simulink model "LMS_cs_old"  (R2023a)
settings: Solver=ode5  StartTime=0.0  StopTime=inf  FixedStep=1/200  RelTol=1e-3
PreLoadFcn:
  | mbxruntime.callbacks.PreLoadFcn(bdroot);
PostLoadFcn:
  | mbxruntime.callbacks.PostLoadFcn(bdroot);
InitFcn:
  | mbxruntime.callbacks.InitFcn(bdroot);
StartFcn:
  | mbxruntime.callbacks.StartFcn(bdroot);
StopFcn:
  | mbxruntime.callbacks.StopFcn(bdroot);
model workspace (MAT data in the model file):
  mbox_table : object (value not decoded)
  model_closed = 0
  sim_status = 0
undefined symbols (not defined in the file or in its folder): DiscIntNeverNeededParam, WheelL0, WheelL1, WheelR0, WheelR1
libraries: simulink x462, simulink_extras x117, PreScanSimulinkLibrary x33, PreScanUsefulBlocks x6, instrumentseriallib x5, simulink_need_slupdate x1
(part 10 of 68)

== system LMS_cs_old/BMW_X5_SUV_4/Dynamics_Simple_3D ==
  DeltaSteer_[deg] : Inport
  Throttle : Inport  Port=2
  Brake : Inport  Port=3
  Initial_Vx_[ms-1] : Inport  Port=4
  AutoManual_OnOff : Inport  Port=5
  Auto_GearShift : Inport  Port=6
  Manual_GearShift : Inport  Port=7
  TyreInfo_in : Inport  Port=8
  Bus Creator : BusCreator  Inputs=14
  Bus Selector : BusSelector  OutputSignals=z_wheelFL_[m],z_wheelFR_[m],z_wheelRL_[m],z_wheelRR_[m]
  Chassis : Subsystem
      mask Display: image(imread('Chassis.png'));
  Engine : Subsystem
      mask Display: image(imread('Engine.png'));
  Gain : Gain  Gain=3.6
  Gear: Auto Manual : Subsystem
  Mux : Mux  Inputs=3
  Radians to Degrees : simulink_extras/Transformations/Radians to Degrees
  Radians to Degrees1 : simulink_extras/Transformations/Radians to Degrees
  Selector : Selector  InputPortWidth=9  IndexOptions=Index vector (dialog)  Indices=7  OutputSizes=1
  Selector1 : Selector  InputPortWidth=9  IndexOptions=Index vector (dialog)  Indices=8  OutputSizes=1
  ShiftLogic : Subsystem
      mask Display: image(imread('Gearshift.png'));
  Transmission : Subsystem
      mask Display: image(imread('Transmission.png'));
  State : Outport
  Vx [m s-1] : Outport  Port=2
  Perf_Params : Outport  Port=3
  z_wheelFL_[m] : Outport  Port=4
  z_wheelFR_[m] : Outport  Port=5
  z_wheelRL_[m] : Outport  Port=6
  z_wheelRR_[m] : Outport  Port=7
  ContactParams : Outport  Port=8
  wires:
  [ax] -> Bus Creator/4  "Ax_[ms-2]"
  [vx] -> Gain/1
  Selector1/1 -> Radians to Degrees1/1
  Selector/1 -> Radians to Degrees/1
  [PD] -> Bus Creator/10  "PDrive_[kW]"
  Radians to Degrees1/1 -> Bus Creator/12  "Pitch_[deg]"
  Radians to Degrees/1 -> Bus Creator/11  "Roll_[deg]"
  [PE] -> Bus Creator/9  "PEngine_[kW]"
  Bus Creator/1 -> Perf_Params/1
  Engine/2(PEngine_[kW]) -> [PE]
  [brake] -> Bus Creator/8  "Brake_[bar]"
  [throttle] -> Bus Creator/7  "Throttle_[perc]"
  [auto_manual] -> Bus Creator/6  "Auto_Manual_[-]"
  [ay] -> Bus Creator/5  "Ay_[ms-2]"
  [gear] -> Bus Creator/3  "Gear_[-]"
  [RPM] -> Bus Creator/2  "NEngine_[rpm]"
  Gain/1 -> Bus Creator/1  "Vx_[kmh-1]"
  Transmission/1(ImpellerTorque_[Nm]) -> Engine/1(ImpellerTorque_[Nm])  "ImpellerTorque_[Nm]"
  Transmission/2(TransmissionTorque_[Nm]) -> Chassis/1(TransmissionTorque_[Nm])  "TransmissionTorque_[Nm]"
  ShiftLogic/1(GearNr) -> ShiftLogic/2(GearNr_[-]), Gear: Auto Manual/3(Auto_Gear)  "GearNr_[-]"
  Engine/1(nEngine_[rpm]) -> Transmission/1(nEngine_[rpm]), [RPM]  "nEngine_[rpm]"
  Chassis/1(State) -> Selector1/1, Selector/1, State/1, Mux/1
  DeltaSteer_[deg]/1 -> Chassis/3(DeltaSteer_[deg])
  Initial_Vx_[ms-1]/1 -> Chassis/4(Initial_Vx_[ms-1])
  Throttle/1 -> [throttle], ShiftLogic/1(Throttle_[%]), Engine/2(Throttle_[%])
  Auto_GearShift/1 -> ShiftLogic/3(Auto_GearShift)
  Chassis/7(TransmissionOut_[rpm]) -> Transmission/3(n_TransmissionOut_[rpm])  "n_driveline_[rpm]"
  Chassis/2(VehicleSpeed_[ms-1]) -> [vx], Vx [m s-1]/1, Mux/2  "vx_[ms-1]"
  AutoManual_OnOff/1 -> [auto_manual], Gear: Auto Manual/1(Auto_Manual)
  Manual_GearShift/1 -> Gear: Auto Manual/2(Manual_Gear)
  Gear: Auto Manual/1(Gear) -> [gear], Transmission/2(GearNr_[-])  "gear"
  [vx] -> ShiftLogic/4(VehSpeed_[ms-1])
  TyreInfo_in/1 -> Chassis/5(TyreInfo_in)
  Brake/1 -> Chassis/2(BrakePressure_[bar]), [brake]
  Chassis/6(PDrive_[kW]) -> [PD]
  Chassis/5(ay_[ms-2]) -> [ay]
  Chassis/4(ax_[ms-2]) -> [ax]
  Chassis/3(Vy_[ms-1]) -> [vy]
  [vx] -> Bus Creator/13  "vx_[ms-1]"
  [vy] -> Bus Creator/14  "vy_[ms-1]"
  Chassis/8(z_wheel_[m]) -> Bus Selector/1, Mux/3  "z_wheel_[m]"
  Bus Selector/1 -> z_wheelFL_[m]/1  "<z_wheelFL_[m]>"
  Bus Selector/2 -> z_wheelFR_[m]/1  "<z_wheelFR_[m]>"
  Bus Selector/3 -> z_wheelRL_[m]/1  "<z_wheelRL_[m]>"
  Bus Selector/4 -> z_wheelRR_[m]/1  "<z_wheelRR_[m]>"
  Mux/1 -> ContactParams/1

== system LMS_cs_old/BMW_X5_SUV_4/JointGroup_WheelDisplacement_V2R ==
  Velocity [m/s] : Inport  SampleTime=TimeStep
  Discrete-Time Integrator : DiscreteIntegrator  SampleTime=TimeStep  ICPrevOutput=DiscIntNeverNeededParam  ICPrevScaledInput=DiscIntNeverNeededParam
  omega=V/Rwheel : Gain  Gain=1/TireRadius
  Rotation [rad] : Outport
  wires:
  Discrete-Time Integrator/1 -> Rotation [rad]/1  "roty"
  omega=V/Rwheel/1 -> Discrete-Time Integrator/1  "rotational speed [rad/s]"
  Velocity [m/s]/1 -> omega=V/Rwheel/1

== system LMS_cs_old/BMW_X5_SUV_4/PreScan_Contact_Sensor ==
  ContactParams : Inport  SampleTime=TimeStep
  Steer Angle Front [deg] : Inport  Port=2
  Steer Angle Rear [deg] : Inport  Port=3
  Bus Creator2 : BusCreator  Inputs=4
  Demux : Demux
  Demux1 : Demux  Outputs=[9 1 4]
  Demux2 : Demux
  For All Wheel Contacts : Subsystem  TreatAsAtomicUnit=on
  Mux6 : Mux  Inputs=2
  Subsystem : Subsystem  mask{NumberOfWheels=4, MaxContactPoints=4, WheelRadius=wheelRadius, WheelWidth=0.2}
      mask prompts: NumberOfWheels "Number of Wheels"; MaxContactPoints "Maximum number of Contact Points"; WheelRadius "Wheel Radius"; WheelWidth "Wheel Width"
      mask Display: disp('Contact Sensor')
  Tire Collision Demux : Subsystem
  Tire Collision Demux1 : Subsystem
  Tire Collision Demux2 : Subsystem
  Tire Collision Demux3 : Subsystem
  Vehicle Local to World : Subsystem
  Wheels = 4 : Subsystem  mask{NumberOfWheels=4}
      mask prompts: NumberOfWheels "Number of Wheels"
      mask Display:
      | port_label('input', 1,'Vehicle wrt World')
      | port_label('input', 2,'Wheels wrt World')
  Wheels Local to World : Subsystem  Tag=MuxWheels  mask(PreScan Mux Block:){}
      settings: DeleteFcn=PreScanBlockDeleteFcn;
  Results : Outport
  wires:
  Mux6/1 -> Wheels = 4/1(Vehicle wrt World)
  Wheels = 4/1(WheelPoses) -> Subsystem/1(In1)
  Demux/1 -> Tire Collision Demux/1(demux in)
  Demux/2 -> Tire Collision Demux1/1(demux in)
  Demux/3 -> Tire Collision Demux2/1(demux in)
  Demux/4 -> Tire Collision Demux3/1(demux in)
  Tire Collision Demux/1(bus out) -> Bus Creator2/1  "TireFL"
  Tire Collision Demux1/1(bus out) -> Bus Creator2/2  "TireFR"
  Tire Collision Demux2/1(bus out) -> Bus Creator2/3  "TireRL"
  Tire Collision Demux3/1(bus out) -> Bus Creator2/4  "TireRR"
  Vehicle Local to World/1(Position) -> Mux6/1
  Vehicle Local to World/2(Orientation) -> Mux6/2
  Wheels Local to World/1(Wheel Poses) -> Wheels = 4/2(Wheels wrt World)
  Demux1/2 -> Wheels Local to World/3(Velocity [m/s])
  Demux2/1 -> Wheels Local to World/4(zDisp FL [m])
  Demux2/2 -> Wheels Local to World/5(zDisp FR [m])
  Demux2/3 -> Wheels Local to World/6(zDisp RL [m])
  Demux2/4 -> Wheels Local to World/7(zDisp RR [m])
  Steer Angle Front [deg]/1 -> Wheels Local to World/1(Steer Angle Front [deg])
  Steer Angle Rear [deg]/1 -> Wheels Local to World/2(Steer Angle Rear [deg])
  Bus Creator2/1 -> Results/1
  ContactParams/1 -> Demux1/1
  Demux1/1 -> Vehicle Local to World/1(State)
  Demux1/3 -> Demux2/1
  Subsystem/1(Out1) -> For All Wheel Contacts/1(In1)
  For All Wheel Contacts/1(Out1) -> Demux/1

== system LMS_cs_old/BMW_X5_SUV_4/SELF_Demux ==
  SELF : Inport  OutDataTypeStr=Bus: PRESCAN_SELFSENSORDATA
  Bus Selector : BusSelector  OutputSignals=PositionX,PositionY,PositionZ,OrientationRoll,OrientationPitch,OrientationYaw,Velocity,Yaw_rate,Lat,Long,Alt
  Demux2 : Demux  Outputs=3
  Gain : Gain  Gain=180/pi
  Gain1 : Gain  Gain=180/pi
  Vector Concatenate1 : Concatenate  NumInputs=3
  compas converter : Subsystem
  x [m] : Outport
  y [m] : Outport  Port=2
  z [m] : Outport  Port=3
  rotx [deg] : Outport  Port=4
  roty [deg] : Outport  Port=5
  rotz [deg] : Outport  Port=6
  GPS lat [deg] : Outport  Port=7
  GPS long [deg] : Outport  Port=8
  GPS alt [m] : Outport  Port=9
  velocity [m/s] : Outport  Port=10
  heading [deg] : Outport  Port=11
  yaw rate [deg/s] : Outport  Port=12
  wires:
  Bus Selector/11 -> GPS alt [m]/1  "<Alt>"
  Bus Selector/10 -> GPS long [deg]/1  "<Long>"
  Bus Selector/9 -> GPS lat [deg]/1  "<Lat>"
  Bus Selector/8 -> Gain1/1  "<Yaw_rate>"
  Bus Selector/7 -> velocity [m/s]/1  "<Velocity>"
  Bus Selector/6 -> compas converter/1(rotz [rad]), Vector Concatenate1/3  "<OrientationYaw>"
  Bus Selector/5 -> Vector Concatenate1/2  "<OrientationPitch>"
  Bus Selector/4 -> Vector Concatenate1/1  "<OrientationRoll>"
  Vector Concatenate1/1 -> Gain/1
  Bus Selector/3 -> z [m]/1  "<PositionZ>"
  Bus Selector/2 -> y [m]/1  "<PositionY>"
  Bus Selector/1 -> x [m]/1  "<PositionX>"
  SELF/1 -> Bus Selector/1
  Gain/1 -> Demux2/1
  Demux2/1 -> rotx [deg]/1
  Demux2/2 -> roty [deg]/1
  Demux2/3 -> rotz [deg]/1
  compas converter/1(heading [deg]) -> heading [deg]/1
  Gain1/1 -> yaw rate [deg/s]/1

== system LMS_cs_old/BMW_X5_SUV_4/STATE_BMW_X5_SUV_4 ==
  State : Inport  SampleTime=TimeStep
  Bus Creator : BusCreator  Inputs=15  OutDataTypeStr=Bus: PRESCAN_STATEACTUATORDATA  NonVirtualBus=on
  Demux : Demux  Outputs=15
  iniBODYAngles wrtVEH [rad] : Constant  Value=[Roll0 Pitch0 0]  SampleTime=TimeStep
  iniVEHAngles wrtGLOB [rad] : Constant  Value=[0 0 Yaw0]  SampleTime=TimeStep
  iniVEHposition wrtGLOB [m] : Constant  Value=[x0 y0 z0]  SampleTime=TimeStep
  state2FullState : PreScanSimulinkLibrary/state2FullState  SystemSampleTime=-1  VariantActivationTime=update diagram  Latency=0  AutoFrameSizeCalculation=off
  StateBus : Outport  OutDataTypeStr=Bus: PRESCAN_STATEACTUATORDATA
  wires:
  Bus Creator/1 -> StateBus/1
  State/1 -> state2FullState/1
  state2FullState/1 -> Demux/1
  iniVEHposition wrtGLOB [m]/1 -> state2FullState/2
  iniBODYAngles wrtVEH [rad]/1 -> state2FullState/3
  iniVEHAngles wrtGLOB [rad]/1 -> state2FullState/4
  Demux/1 -> Bus Creator/1  "PositionX"
  Demux/2 -> Bus Creator/2  "PositionY"
  Demux/3 -> Bus Creator/3  "PositionZ"
  Demux/4 -> Bus Creator/4  "VelocityX"
  Demux/5 -> Bus Creator/5  "VelocityY"
  Demux/6 -> Bus Creator/6  "VelocityZ"
  Demux/7 -> Bus Creator/7  "AccelerationX"
  Demux/8 -> Bus Creator/8  "AccelerationY"
  Demux/9 -> Bus Creator/9  "AccelerationZ"
  Demux/10 -> Bus Creator/10  "OrientationRoll"
  Demux/11 -> Bus Creator/11  "OrientationPitch"
  Demux/12 -> Bus Creator/12  "OrientationYaw"
  Demux/13 -> Bus Creator/13  "AngularVelocityRoll"
  Demux/14 -> Bus Creator/14  "AngularVelocityPitch"
  Demux/15 -> Bus Creator/15  "AngularVelocityYaw"

== system LMS_cs_old/BMW_X5_SUV_4/WheelDisplacement_Mux ==
  Steering Angle Front [rad] : Inport  Tag=inport/JointGroup  SampleTime=2/200  BusOutputAsStruct=on
  Steering Angle Rear [rad] : Inport  Tag=inport/JointGroup  Port=2  SampleTime=2/200  BusOutputAsStruct=on
  Rotation [rad] : Inport  Tag=inport/JointGroup  Port=3  SampleTime=2/200  BusOutputAsStruct=on
  zDisp FL [m] : Inport  Tag=inport/JointGroup  Port=4  SampleTime=2/200  BusOutputAsStruct=on
  zDisp FR [m] : Inport  Tag=inport/JointGroup  Port=5  SampleTime=2/200  BusOutputAsStruct=on
  zDisp RL [m] : Inport  Tag=inport/JointGroup  Port=6  SampleTime=2/200  BusOutputAsStruct=on
  zDisp RR [m] : Inport  Tag=inport/JointGroup  Port=7  SampleTime=2/200  BusOutputAsStruct=on
  Ground_{1..12} (12 alike) : Ground
  WheelL0_Mux : Subsystem  Tag=mux/Joint  mask(PreScan Mux Block){DisplayName=WheelL0}
      mask prompts: DisplayName "Display Name"
      mask help:
      | This block simulates a generic joint used for generic models. This joint can be enabled/disabled from the GUI.
      |
      | For more information, please click Help.
      settings: DeleteFcn=PreScanBlockDeleteFcn;
      mask Help: eval('openHelp(254)')
  WheelL1_Mux : Subsystem  Tag=mux/Joint  mask(PreScan Mux Block){DisplayName=WheelL1}
      mask prompts: DisplayName "Display Name"
      mask help:
      | This block simulates a generic joint used for generic models. This joint can be enabled/disabled from the GUI.
      |
      | For more information, please click Help.
      settings: DeleteFcn=PreScanBlockDeleteFcn;
      mask Help: eval('openHelp(254)')
  WheelR0_Mux : Subsystem  Tag=mux/Joint  mask(PreScan Mux Block){DisplayName=WheelR0}
      mask prompts: DisplayName "Display Name"
      mask help:
      | This block simulates a generic joint used for generic models. This joint can be enabled/disabled from the GUI.
      |
      | For more information, please click Help.
      settings: DeleteFcn=PreScanBlockDeleteFcn;
      mask Help: eval('openHelp(254)')
  WheelR1_Mux : Subsystem  Tag=mux/Joint  mask(PreScan Mux Block){DisplayName=WheelR1}
      mask prompts: DisplayName "Display Name"
      mask help:
      | This block simulates a generic joint used for generic models. This joint can be enabled/disabled from the GUI.
      |
      | For more information, please click Help.
      settings: DeleteFcn=PreScanBlockDeleteFcn;
      mask Help: eval('openHelp(254)')
  WheelL0_BMW_X5_SUV_4 : Outport  Tag=outport/JointActuator  OutDataTypeStr=Bus: PRESCAN_POSE_DATA  SampleTime=2/200
  WheelR0_BMW_X5_SUV_4 : Outport  Tag=outport/JointActuator  Port=2  OutDataTypeStr=Bus: PRESCAN_POSE_DATA  SampleTime=2/200
  WheelR1_BMW_X5_SUV_4 : Outport  Tag=outport/JointActuator  Port=3  OutDataTypeStr=Bus: PRESCAN_POSE_DATA  SampleTime=2/200
  WheelL1_BMW_X5_SUV_4 : Outport  Tag=outport/JointActuator  Port=4  OutDataTypeStr=Bus: PRESCAN_POSE_DATA  SampleTime=2/200
  wires:
  WheelL0_Mux/1(Joint) -> WheelL0_BMW_X5_SUV_4/1
  WheelR0_Mux/1(Joint) -> WheelR0_BMW_X5_SUV_4/1
  WheelR1_Mux/1(Joint) -> WheelR1_BMW_X5_SUV_4/1
  WheelL1_Mux/1(Joint) -> WheelL1_BMW_X5_SUV_4/1
  Steering Angle Front [rad]/1 -> WheelR0_Mux/6(Yaw [rad]), WheelL0_Mux/6(Yaw [rad])
  Steering Angle Rear [rad]/1 -> WheelR1_Mux/6(Yaw [rad]), WheelL1_Mux/6(Yaw [rad])
  Rotation [rad]/1 -> WheelR0_Mux/5(Pitch [rad]), WheelL0_Mux/5(Pitch [rad]), WheelR1_Mux/5(Pitch [rad]), WheelL1_Mux/5(Pitch [rad])
  zDisp FL [m]/1 -> WheelL0_Mux/3(Z [m])
  zDisp FR [m]/1 -> WheelR0_Mux/3(Z [m])
  zDisp RL [m]/1 -> WheelL1_Mux/3(Z [m])
  zDisp RR [m]/1 -> WheelR1_Mux/3(Z [m])
  Ground_1/1 -> WheelL0_Mux/1(X [m])
  Ground_2/1 -> WheelL0_Mux/2(Y [m])
  Ground_3/1 -> WheelL0_Mux/4(Roll [rad])
  Ground_4/1 -> WheelL1_Mux/1(X [m])
  Ground_5/1 -> WheelL1_Mux/2(Y [m])
  Ground_6/1 -> WheelL1_Mux/4(Roll [rad])
  Ground_7/1 -> WheelR0_Mux/1(X [m])
  Ground_8/1 -> WheelR0_Mux/2(Y [m])
  Ground_9/1 -> WheelR0_Mux/4(Roll [rad])
  Ground_10/1 -> WheelR1_Mux/1(X [m])
  Ground_11/1 -> WheelR1_Mux/2(Y [m])
  Ground_12/1 -> WheelR1_Mux/4(Roll [rad])

== system LMS_cs_old/BMW_X5_SUV_5/Dynamics_Simple_3D ==
  DeltaSteer_[deg] : Inport
  Throttle : Inport  Port=2
  Brake : Inport  Port=3
  Initial_Vx_[ms-1] : Inport  Port=4
  AutoManual_OnOff : Inport  Port=5
  Auto_GearShift : Inport  Port=6
  Manual_GearShift : Inport  Port=7
  TyreInfo_in : Inport  Port=8
  Bus Creator : BusCreator  Inputs=14
  Bus Selector : BusSelector  OutputSignals=z_wheelFL_[m],z_wheelFR_[m],z_wheelRL_[m],z_wheelRR_[m]
  Chassis : Subsystem
      mask Display: image(imread('Chassis.png'));
  Engine : Subsystem
      mask Display: image(imread('Engine.png'));
  Gain : Gain  Gain=3.6
  Gear: Auto Manual : Subsystem
  Mux : Mux  Inputs=3
  Radians to Degrees : simulink_extras/Transformations/Radians to Degrees
  Radians to Degrees1 : simulink_extras/Transformations/Radians to Degrees
  Selector : Selector  InputPortWidth=9  IndexOptions=Index vector (dialog)  Indices=7  OutputSizes=1
  Selector1 : Selector  InputPortWidth=9  IndexOptions=Index vector (dialog)  Indices=8  OutputSizes=1
  ShiftLogic : Subsystem
      mask Display: image(imread('Gearshift.png'));
  Transmission : Subsystem
      mask Display: image(imread('Transmission.png'));
  State : Outport
  Vx [m s-1] : Outport  Port=2
  Perf_Params : Outport  Port=3
  z_wheelFL_[m] : Outport  Port=4
  z_wheelFR_[m] : Outport  Port=5
  z_wheelRL_[m] : Outport  Port=6
  z_wheelRR_[m] : Outport  Port=7
  ContactParams : Outport  Port=8
  wires:
  [ax] -> Bus Creator/4  "Ax_[ms-2]"
  [vx] -> Gain/1
  Selector1/1 -> Radians to Degrees1/1
  Selector/1 -> Radians to Degrees/1
  [PD] -> Bus Creator/10  "PDrive_[kW]"
  Radians to Degrees1/1 -> Bus Creator/12  "Pitch_[deg]"
  Radians to Degrees/1 -> Bus Creator/11  "Roll_[deg]"
  [PE] -> Bus Creator/9  "PEngine_[kW]"
  Bus Creator/1 -> Perf_Params/1
  Engine/2(PEngine_[kW]) -> [PE]
  [brake] -> Bus Creator/8  "Brake_[bar]"
  [throttle] -> Bus Creator/7  "Throttle_[perc]"
  [auto_manual] -> Bus Creator/6  "Auto_Manual_[-]"
  [ay] -> Bus Creator/5  "Ay_[ms-2]"
  [gear] -> Bus Creator/3  "Gear_[-]"
  [RPM] -> Bus Creator/2  "NEngine_[rpm]"
  Gain/1 -> Bus Creator/1  "Vx_[kmh-1]"
  Transmission/1(ImpellerTorque_[Nm]) -> Engine/1(ImpellerTorque_[Nm])  "ImpellerTorque_[Nm]"
  Transmission/2(TransmissionTorque_[Nm]) -> Chassis/1(TransmissionTorque_[Nm])  "TransmissionTorque_[Nm]"
  ShiftLogic/1(GearNr) -> ShiftLogic/2(GearNr_[-]), Gear: Auto Manual/3(Auto_Gear)  "GearNr_[-]"
  Engine/1(nEngine_[rpm]) -> Transmission/1(nEngine_[rpm]), [RPM]  "nEngine_[rpm]"
  Chassis/1(State) -> Selector1/1, Selector/1, State/1, Mux/1
  DeltaSteer_[deg]/1 -> Chassis/3(DeltaSteer_[deg])
  Initial_Vx_[ms-1]/1 -> Chassis/4(Initial_Vx_[ms-1])
  Throttle/1 -> [throttle], ShiftLogic/1(Throttle_[%]), Engine/2(Throttle_[%])
  Auto_GearShift/1 -> ShiftLogic/3(Auto_GearShift)
  Chassis/7(TransmissionOut_[rpm]) -> Transmission/3(n_TransmissionOut_[rpm])  "n_driveline_[rpm]"
  Chassis/2(VehicleSpeed_[ms-1]) -> [vx], Vx [m s-1]/1, Mux/2  "vx_[ms-1]"
  AutoManual_OnOff/1 -> [auto_manual], Gear: Auto Manual/1(Auto_Manual)
  Manual_GearShift/1 -> Gear: Auto Manual/2(Manual_Gear)
  Gear: Auto Manual/1(Gear) -> [gear], Transmission/2(GearNr_[-])  "gear"
  [vx] -> ShiftLogic/4(VehSpeed_[ms-1])
  TyreInfo_in/1 -> Chassis/5(TyreInfo_in)
  Brake/1 -> Chassis/2(BrakePressure_[bar]), [brake]
  Chassis/6(PDrive_[kW]) -> [PD]
  Chassis/5(ay_[ms-2]) -> [ay]
  Chassis/4(ax_[ms-2]) -> [ax]
  Chassis/3(Vy_[ms-1]) -> [vy]
  [vx] -> Bus Creator/13  "vx_[ms-1]"
  [vy] -> Bus Creator/14  "vy_[ms-1]"
  Chassis/8(z_wheel_[m]) -> Bus Selector/1, Mux/3  "z_wheel_[m]"
  Bus Selector/1 -> z_wheelFL_[m]/1  "<z_wheelFL_[m]>"
  Bus Selector/2 -> z_wheelFR_[m]/1  "<z_wheelFR_[m]>"
  Bus Selector/3 -> z_wheelRL_[m]/1  "<z_wheelRL_[m]>"
  Bus Selector/4 -> z_wheelRR_[m]/1  "<z_wheelRR_[m]>"
  Mux/1 -> ContactParams/1

== system LMS_cs_old/BMW_X5_SUV_5/JointGroup_WheelDisplacement_V2R ==
  Velocity [m/s] : Inport  SampleTime=TimeStep
  Discrete-Time Integrator : DiscreteIntegrator  SampleTime=TimeStep  ICPrevOutput=DiscIntNeverNeededParam  ICPrevScaledInput=DiscIntNeverNeededParam
  omega=V/Rwheel : Gain  Gain=1/TireRadius
  Rotation [rad] : Outport
  wires:
  Discrete-Time Integrator/1 -> Rotation [rad]/1  "roty"
  omega=V/Rwheel/1 -> Discrete-Time Integrator/1  "rotational speed [rad/s]"
  Velocity [m/s]/1 -> omega=V/Rwheel/1

== system LMS_cs_old/BMW_X5_SUV_5/PreScan_Contact_Sensor ==
  ContactParams : Inport  SampleTime=TimeStep
  Steer Angle Front [deg] : Inport  Port=2
  Steer Angle Rear [deg] : Inport  Port=3
  Bus Creator2 : BusCreator  Inputs=4
  Demux : Demux
  Demux1 : Demux  Outputs=[9 1 4]
  Demux2 : Demux
  For All Wheel Contacts : Subsystem  TreatAsAtomicUnit=on
  Mux6 : Mux  Inputs=2
  Subsystem : Subsystem  mask{NumberOfWheels=4, MaxContactPoints=4, WheelRadius=wheelRadius, WheelWidth=0.2}
      mask prompts: NumberOfWheels "Number of Wheels"; MaxContactPoints "Maximum number of Contact Points"; WheelRadius "Wheel Radius"; WheelWidth "Wheel Width"
      mask Display: disp('Contact Sensor')
  Tire Collision Demux : Subsystem
  Tire Collision Demux1 : Subsystem
  Tire Collision Demux2 : Subsystem
  Tire Collision Demux3 : Subsystem
  Vehicle Local to World : Subsystem
  Wheels = 4 : Subsystem  mask{NumberOfWheels=4}
      mask prompts: NumberOfWheels "Number of Wheels"
      mask Display:
      | port_label('input', 1,'Vehicle wrt World')
      | port_label('input', 2,'Wheels wrt World')
  Wheels Local to World : Subsystem  Tag=MuxWheels  mask(PreScan Mux Block:){}
      settings: DeleteFcn=PreScanBlockDeleteFcn;
  Results : Outport
  wires:
  Mux6/1 -> Wheels = 4/1(Vehicle wrt World)
  Wheels = 4/1(WheelPoses) -> Subsystem/1(In1)
  Demux/1 -> Tire Collision Demux/1(demux in)
  Demux/2 -> Tire Collision Demux1/1(demux in)
  Demux/3 -> Tire Collision Demux2/1(demux in)
  Demux/4 -> Tire Collision Demux3/1(demux in)
  Tire Collision Demux/1(bus out) -> Bus Creator2/1  "TireFL"
  Tire Collision Demux1/1(bus out) -> Bus Creator2/2  "TireFR"
  Tire Collision Demux2/1(bus out) -> Bus Creator2/3  "TireRL"
  Tire Collision Demux3/1(bus out) -> Bus Creator2/4  "TireRR"
  Vehicle Local to World/1(Position) -> Mux6/1
  Vehicle Local to World/2(Orientation) -> Mux6/2
  Wheels Local to World/1(Wheel Poses) -> Wheels = 4/2(Wheels wrt World)
  Demux1/2 -> Wheels Local to World/3(Velocity [m/s])
  Demux2/1 -> Wheels Local to World/4(zDisp FL [m])
  Demux2/2 -> Wheels Local to World/5(zDisp FR [m])
  Demux2/3 -> Wheels Local to World/6(zDisp RL [m])
  Demux2/4 -> Wheels Local to World/7(zDisp RR [m])
  Steer Angle Front [deg]/1 -> Wheels Local to World/1(Steer Angle Front [deg])
  Steer Angle Rear [deg]/1 -> Wheels Local to World/2(Steer Angle Rear [deg])
  Bus Creator2/1 -> Results/1
  ContactParams/1 -> Demux1/1
  Demux1/1 -> Vehicle Local to World/1(State)
  Demux1/3 -> Demux2/1
  Subsystem/1(Out1) -> For All Wheel Contacts/1(In1)
  For All Wheel Contacts/1(Out1) -> Demux/1

== system LMS_cs_old/BMW_X5_SUV_5/SELF_Demux ==
  SELF : Inport  OutDataTypeStr=Bus: PRESCAN_SELFSENSORDATA
  Bus Selector : BusSelector  OutputSignals=PositionX,PositionY,PositionZ,OrientationRoll,OrientationPitch,OrientationYaw,Velocity,Yaw_rate,Lat,Long,Alt
  Demux2 : Demux  Outputs=3
  Gain : Gain  Gain=180/pi
  Gain1 : Gain  Gain=180/pi
  Vector Concatenate1 : Concatenate  NumInputs=3
  compas converter : Subsystem
  x [m] : Outport
  y [m] : Outport  Port=2
  z [m] : Outport  Port=3
  rotx [deg] : Outport  Port=4
  roty [deg] : Outport  Port=5
  rotz [deg] : Outport  Port=6
  GPS lat [deg] : Outport  Port=7
  GPS long [deg] : Outport  Port=8
  GPS alt [m] : Outport  Port=9
  velocity [m/s] : Outport  Port=10
  heading [deg] : Outport  Port=11
  yaw rate [deg/s] : Outport  Port=12
  wires:
  Bus Selector/11 -> GPS alt [m]/1  "<Alt>"
  Bus Selector/10 -> GPS long [deg]/1  "<Long>"
  Bus Selector/9 -> GPS lat [deg]/1  "<Lat>"
  Bus Selector/8 -> Gain1/1  "<Yaw_rate>"
  Bus Selector/7 -> velocity [m/s]/1  "<Velocity>"
  Bus Selector/6 -> compas converter/1(rotz [rad]), Vector Concatenate1/3  "<OrientationYaw>"
  Bus Selector/5 -> Vector Concatenate1/2  "<OrientationPitch>"
  Bus Selector/4 -> Vector Concatenate1/1  "<OrientationRoll>"
  Vector Concatenate1/1 -> Gain/1
  Bus Selector/3 -> z [m]/1  "<PositionZ>"
  Bus Selector/2 -> y [m]/1  "<PositionY>"
  Bus Selector/1 -> x [m]/1  "<PositionX>"
  SELF/1 -> Bus Selector/1
  Gain/1 -> Demux2/1
  Demux2/1 -> rotx [deg]/1
  Demux2/2 -> roty [deg]/1
  Demux2/3 -> rotz [deg]/1
  compas converter/1(heading [deg]) -> heading [deg]/1
  Gain1/1 -> yaw rate [deg/s]/1

== system LMS_cs_old/BMW_X5_SUV_5/STATE_BMW_X5_SUV_5 ==
  State : Inport  SampleTime=TimeStep
  Bus Creator : BusCreator  Inputs=15  OutDataTypeStr=Bus: PRESCAN_STATEACTUATORDATA  NonVirtualBus=on
  Demux : Demux  Outputs=15
  iniBODYAngles wrtVEH [rad] : Constant  Value=[Roll0 Pitch0 0]  SampleTime=TimeStep
  iniVEHAngles wrtGLOB [rad] : Constant  Value=[0 0 Yaw0]  SampleTime=TimeStep
  iniVEHposition wrtGLOB [m] : Constant  Value=[x0 y0 z0]  SampleTime=TimeStep
  state2FullState : PreScanSimulinkLibrary/state2FullState  SystemSampleTime=-1  VariantActivationTime=update diagram  Latency=0  AutoFrameSizeCalculation=off
  StateBus : Outport  OutDataTypeStr=Bus: PRESCAN_STATEACTUATORDATA
  wires:
  Bus Creator/1 -> StateBus/1
  State/1 -> state2FullState/1
  state2FullState/1 -> Demux/1
  iniVEHposition wrtGLOB [m]/1 -> state2FullState/2
  iniBODYAngles wrtVEH [rad]/1 -> state2FullState/3
  iniVEHAngles wrtGLOB [rad]/1 -> state2FullState/4
  Demux/1 -> Bus Creator/1  "PositionX"
  Demux/2 -> Bus Creator/2  "PositionY"
  Demux/3 -> Bus Creator/3  "PositionZ"
  Demux/4 -> Bus Creator/4  "VelocityX"
  Demux/5 -> Bus Creator/5  "VelocityY"
  Demux/6 -> Bus Creator/6  "VelocityZ"
  Demux/7 -> Bus Creator/7  "AccelerationX"
  Demux/8 -> Bus Creator/8  "AccelerationY"
  Demux/9 -> Bus Creator/9  "AccelerationZ"
  Demux/10 -> Bus Creator/10  "OrientationRoll"
  Demux/11 -> Bus Creator/11  "OrientationPitch"
  Demux/12 -> Bus Creator/12  "OrientationYaw"
  Demux/13 -> Bus Creator/13  "AngularVelocityRoll"
  Demux/14 -> Bus Creator/14  "AngularVelocityPitch"
  Demux/15 -> Bus Creator/15  "AngularVelocityYaw"

== system LMS_cs_old/BMW_X5_SUV_5/WheelDisplacement_Mux ==
  Steering Angle Front [rad] : Inport  Tag=inport/JointGroup  SampleTime=2/200  BusOutputAsStruct=on
  Steering Angle Rear [rad] : Inport  Tag=inport/JointGroup  Port=2  SampleTime=2/200  BusOutputAsStruct=on
  Rotation [rad] : Inport  Tag=inport/JointGroup  Port=3  SampleTime=2/200  BusOutputAsStruct=on
  zDisp FL [m] : Inport  Tag=inport/JointGroup  Port=4  SampleTime=2/200  BusOutputAsStruct=on
  zDisp FR [m] : Inport  Tag=inport/JointGroup  Port=5  SampleTime=2/200  BusOutputAsStruct=on
  zDisp RL [m] : Inport  Tag=inport/JointGroup  Port=6  SampleTime=2/200  BusOutputAsStruct=on
  zDisp RR [m] : Inport  Tag=inport/JointGroup  Port=7  SampleTime=2/200  BusOutputAsStruct=on
  Ground_{1..12} (12 alike) : Ground
  WheelL0_Mux : Subsystem  Tag=mux/Joint  mask(PreScan Mux Block){DisplayName=WheelL0}
      mask prompts: DisplayName "Display Name"
      mask help:
      | This block simulates a generic joint used for generic models. This joint can be enabled/disabled from the GUI.
      |
      | For more information, please click Help.
      settings: DeleteFcn=PreScanBlockDeleteFcn;
      mask Help: eval('openHelp(254)')
  WheelL1_Mux : Subsystem  Tag=mux/Joint  mask(PreScan Mux Block){DisplayName=WheelL1}
      mask prompts: DisplayName "Display Name"
      mask help:
      | This block simulates a generic joint used for generic models. This joint can be enabled/disabled from the GUI.
      |
      | For more information, please click Help.
      settings: DeleteFcn=PreScanBlockDeleteFcn;
      mask Help: eval('openHelp(254)')
  WheelR0_Mux : Subsystem  Tag=mux/Joint  mask(PreScan Mux Block){DisplayName=WheelR0}
      mask prompts: DisplayName "Display Name"
      mask help:
      | This block simulates a generic joint used for generic models. This joint can be enabled/disabled from the GUI.
      |
      | For more information, please click Help.
      settings: DeleteFcn=PreScanBlockDeleteFcn;
      mask Help: eval('openHelp(254)')
  WheelR1_Mux : Subsystem  Tag=mux/Joint  mask(PreScan Mux Block){DisplayName=WheelR1}
      mask prompts: DisplayName "Display Name"
      mask help:
      | This block simulates a generic joint used for generic models. This joint can be enabled/disabled from the GUI.
      |
      | For more information, please click Help.
      settings: DeleteFcn=PreScanBlockDeleteFcn;
      mask Help: eval('openHelp(254)')
  WheelL0_BMW_X5_SUV_5 : Outport  Tag=outport/JointActuator  OutDataTypeStr=Bus: PRESCAN_POSE_DATA  SampleTime=2/200
  WheelR0_BMW_X5_SUV_5 : Outport  Tag=outport/JointActuator  Port=2  OutDataTypeStr=Bus: PRESCAN_POSE_DATA  SampleTime=2/200
  WheelR1_BMW_X5_SUV_5 : Outport  Tag=outport/JointActuator  Port=3  OutDataTypeStr=Bus: PRESCAN_POSE_DATA  SampleTime=2/200
  WheelL1_BMW_X5_SUV_5 : Outport  Tag=outport/JointActuator  Port=4  OutDataTypeStr=Bus: PRESCAN_POSE_DATA  SampleTime=2/200
  wires:
  WheelL0_Mux/1(Joint) -> WheelL0_BMW_X5_SUV_5/1
  WheelR0_Mux/1(Joint) -> WheelR0_BMW_X5_SUV_5/1
  WheelR1_Mux/1(Joint) -> WheelR1_BMW_X5_SUV_5/1
  WheelL1_Mux/1(Joint) -> WheelL1_BMW_X5_SUV_5/1
  Steering Angle Front [rad]/1 -> WheelR0_Mux/6(Yaw [rad]), WheelL0_Mux/6(Yaw [rad])
  Steering Angle Rear [rad]/1 -> WheelR1_Mux/6(Yaw [rad]), WheelL1_Mux/6(Yaw [rad])
  Rotation [rad]/1 -> WheelR0_Mux/5(Pitch [rad]), WheelL0_Mux/5(Pitch [rad]), WheelR1_Mux/5(Pitch [rad]), WheelL1_Mux/5(Pitch [rad])
  zDisp FL [m]/1 -> WheelL0_Mux/3(Z [m])
  zDisp FR [m]/1 -> WheelR0_Mux/3(Z [m])
  zDisp RL [m]/1 -> WheelL1_Mux/3(Z [m])
  zDisp RR [m]/1 -> WheelR1_Mux/3(Z [m])
  Ground_1/1 -> WheelL0_Mux/1(X [m])
  Ground_2/1 -> WheelL0_Mux/2(Y [m])
  Ground_3/1 -> WheelL0_Mux/4(Roll [rad])
  Ground_4/1 -> WheelL1_Mux/1(X [m])
  Ground_5/1 -> WheelL1_Mux/2(Y [m])
  Ground_6/1 -> WheelL1_Mux/4(Roll [rad])
  Ground_7/1 -> WheelR0_Mux/1(X [m])
  Ground_8/1 -> WheelR0_Mux/2(Y [m])
  Ground_9/1 -> WheelR0_Mux/4(Roll [rad])
  Ground_10/1 -> WheelR1_Mux/1(X [m])
  Ground_11/1 -> WheelR1_Mux/2(Y [m])
  Ground_12/1 -> WheelR1_Mux/4(Roll [rad])

== system LMS_cs_old/BMW_X5_SUV_6/Dynamics_Simple_3D ==
  DeltaSteer_[deg] : Inport
  Throttle : Inport  Port=2
  Brake : Inport  Port=3
  Initial_Vx_[ms-1] : Inport  Port=4
  AutoManual_OnOff : Inport  Port=5
  Auto_GearShift : Inport  Port=6
  Manual_GearShift : Inport  Port=7
  TyreInfo_in : Inport  Port=8
  Bus Creator : BusCreator  Inputs=14
  Bus Selector : BusSelector  OutputSignals=z_wheelFL_[m],z_wheelFR_[m],z_wheelRL_[m],z_wheelRR_[m]
  Chassis : Subsystem
      mask Display: image(imread('Chassis.png'));
  Engine : Subsystem
      mask Display: image(imread('Engine.png'));
  Gain : Gain  Gain=3.6
  Gear: Auto Manual : Subsystem
  Mux : Mux  Inputs=3
  Radians to Degrees : simulink_extras/Transformations/Radians to Degrees
  Radians to Degrees1 : simulink_extras/Transformations/Radians to Degrees
  Selector : Selector  InputPortWidth=9  IndexOptions=Index vector (dialog)  Indices=7  OutputSizes=1
  Selector1 : Selector  InputPortWidth=9  IndexOptions=Index vector (dialog)  Indices=8  OutputSizes=1
  ShiftLogic : Subsystem
      mask Display: image(imread('Gearshift.png'));
  Transmission : Subsystem
      mask Display: image(imread('Transmission.png'));
  State : Outport
  Vx [m s-1] : Outport  Port=2
  Perf_Params : Outport  Port=3
  z_wheelFL_[m] : Outport  Port=4
  z_wheelFR_[m] : Outport  Port=5
  z_wheelRL_[m] : Outport  Port=6
  z_wheelRR_[m] : Outport  Port=7
  ContactParams : Outport  Port=8
  wires:
  [ax] -> Bus Creator/4  "Ax_[ms-2]"
  [vx] -> Gain/1
  Selector1/1 -> Radians to Degrees1/1
  Selector/1 -> Radians to Degrees/1
  [PD] -> Bus Creator/10  "PDrive_[kW]"
  Radians to Degrees1/1 -> Bus Creator/12  "Pitch_[deg]"
  Radians to Degrees/1 -> Bus Creator/11  "Roll_[deg]"
  [PE] -> Bus Creator/9  "PEngine_[kW]"
  Bus Creator/1 -> Perf_Params/1
  Engine/2(PEngine_[kW]) -> [PE]
  [brake] -> Bus Creator/8  "Brake_[bar]"
  [throttle] -> Bus Creator/7  "Throttle_[perc]"
  [auto_manual] -> Bus Creator/6  "Auto_Manual_[-]"
  [ay] -> Bus Creator/5  "Ay_[ms-2]"
  [gear] -> Bus Creator/3  "Gear_[-]"
  [RPM] -> Bus Creator/2  "NEngine_[rpm]"
  Gain/1 -> Bus Creator/1  "Vx_[kmh-1]"
  Transmission/1(ImpellerTorque_[Nm]) -> Engine/1(ImpellerTorque_[Nm])  "ImpellerTorque_[Nm]"
  Transmission/2(TransmissionTorque_[Nm]) -> Chassis/1(TransmissionTorque_[Nm])  "TransmissionTorque_[Nm]"
  ShiftLogic/1(GearNr) -> ShiftLogic/2(GearNr_[-]), Gear: Auto Manual/3(Auto_Gear)  "GearNr_[-]"
  Engine/1(nEngine_[rpm]) -> Transmission/1(nEngine_[rpm]), [RPM]  "nEngine_[rpm]"
  Chassis/1(State) -> Selector1/1, Selector/1, State/1, Mux/1
  DeltaSteer_[deg]/1 -> Chassis/3(DeltaSteer_[deg])
  Initial_Vx_[ms-1]/1 -> Chassis/4(Initial_Vx_[ms-1])
  Throttle/1 -> [throttle], ShiftLogic/1(Throttle_[%]), Engine/2(Throttle_[%])
  Auto_GearShift/1 -> ShiftLogic/3(Auto_GearShift)
  Chassis/7(TransmissionOut_[rpm]) -> Transmission/3(n_TransmissionOut_[rpm])  "n_driveline_[rpm]"
  Chassis/2(VehicleSpeed_[ms-1]) -> [vx], Vx [m s-1]/1, Mux/2  "vx_[ms-1]"
  AutoManual_OnOff/1 -> [auto_manual], Gear: Auto Manual/1(Auto_Manual)
  Manual_GearShift/1 -> Gear: Auto Manual/2(Manual_Gear)
  Gear: Auto Manual/1(Gear) -> [gear], Transmission/2(GearNr_[-])  "gear"
  [vx] -> ShiftLogic/4(VehSpeed_[ms-1])
  TyreInfo_in/1 -> Chassis/5(TyreInfo_in)
  Brake/1 -> Chassis/2(BrakePressure_[bar]), [brake]
  Chassis/6(PDrive_[kW]) -> [PD]
  Chassis/5(ay_[ms-2]) -> [ay]
  Chassis/4(ax_[ms-2]) -> [ax]
  Chassis/3(Vy_[ms-1]) -> [vy]
  [vx] -> Bus Creator/13  "vx_[ms-1]"
  [vy] -> Bus Creator/14  "vy_[ms-1]"
  Chassis/8(z_wheel_[m]) -> Bus Selector/1, Mux/3  "z_wheel_[m]"
  Bus Selector/1 -> z_wheelFL_[m]/1  "<z_wheelFL_[m]>"
  Bus Selector/2 -> z_wheelFR_[m]/1  "<z_wheelFR_[m]>"
  Bus Selector/3 -> z_wheelRL_[m]/1  "<z_wheelRL_[m]>"
  Bus Selector/4 -> z_wheelRR_[m]/1  "<z_wheelRR_[m]>"
  Mux/1 -> ContactParams/1

== system LMS_cs_old/BMW_X5_SUV_6/JointGroup_WheelDisplacement_V2R ==
  Velocity [m/s] : Inport  SampleTime=TimeStep
  Discrete-Time Integrator : DiscreteIntegrator  SampleTime=TimeStep  ICPrevOutput=DiscIntNeverNeededParam  ICPrevScaledInput=DiscIntNeverNeededParam
  omega=V/Rwheel : Gain  Gain=1/TireRadius
  Rotation [rad] : Outport
  wires:
  Discrete-Time Integrator/1 -> Rotation [rad]/1  "roty"
  omega=V/Rwheel/1 -> Discrete-Time Integrator/1  "rotational speed [rad/s]"
  Velocity [m/s]/1 -> omega=V/Rwheel/1

== system LMS_cs_old/BMW_X5_SUV_6/PreScan_Contact_Sensor ==
  ContactParams : Inport  SampleTime=TimeStep
  Steer Angle Front [deg] : Inport  Port=2
  Steer Angle Rear [deg] : Inport  Port=3
  Bus Creator2 : BusCreator  Inputs=4
  Demux : Demux
  Demux1 : Demux  Outputs=[9 1 4]
  Demux2 : Demux
  For All Wheel Contacts : Subsystem  TreatAsAtomicUnit=on
  Mux6 : Mux  Inputs=2
  Subsystem : Subsystem  mask{NumberOfWheels=4, MaxContactPoints=4, WheelRadius=wheelRadius, WheelWidth=0.2}
      mask prompts: NumberOfWheels "Number of Wheels"; MaxContactPoints "Maximum number of Contact Points"; WheelRadius "Wheel Radius"; WheelWidth "Wheel Width"
      mask Display: disp('Contact Sensor')
  Tire Collision Demux : Subsystem
  Tire Collision Demux1 : Subsystem
  Tire Collision Demux2 : Subsystem
  Tire Collision Demux3 : Subsystem
  Vehicle Local to World : Subsystem
  Wheels = 4 : Subsystem  mask{NumberOfWheels=4}
      mask prompts: NumberOfWheels "Number of Wheels"
      mask Display:
      | port_label('input', 1,'Vehicle wrt World')
      | port_label('input', 2,'Wheels wrt World')
  Wheels Local to World : Subsystem  Tag=MuxWheels  mask(PreScan Mux Block:){}
      settings: DeleteFcn=PreScanBlockDeleteFcn;
  Results : Outport
  wires:
  Mux6/1 -> Wheels = 4/1(Vehicle wrt World)
  Wheels = 4/1(WheelPoses) -> Subsystem/1(In1)
  Demux/1 -> Tire Collision Demux/1(demux in)
  Demux/2 -> Tire Collision Demux1/1(demux in)
  Demux/3 -> Tire Collision Demux2/1(demux in)
  Demux/4 -> Tire Collision Demux3/1(demux in)
  Tire Collision Demux/1(bus out) -> Bus Creator2/1  "TireFL"
  Tire Collision Demux1/1(bus out) -> Bus Creator2/2  "TireFR"
  Tire Collision Demux2/1(bus out) -> Bus Creator2/3  "TireRL"
  Tire Collision Demux3/1(bus out) -> Bus Creator2/4  "TireRR"
  Vehicle Local to World/1(Position) -> Mux6/1
  Vehicle Local to World/2(Orientation) -> Mux6/2
  Wheels Local to World/1(Wheel Poses) -> Wheels = 4/2(Wheels wrt World)
  Demux1/2 -> Wheels Local to World/3(Velocity [m/s])
  Demux2/1 -> Wheels Local to World/4(zDisp FL [m])
  Demux2/2 -> Wheels Local to World/5(zDisp FR [m])
  Demux2/3 -> Wheels Local to World/6(zDisp RL [m])
  Demux2/4 -> Wheels Local to World/7(zDisp RR [m])
  Steer Angle Front [deg]/1 -> Wheels Local to World/1(Steer Angle Front [deg])
  Steer Angle Rear [deg]/1 -> Wheels Local to World/2(Steer Angle Rear [deg])
  Bus Creator2/1 -> Results/1
  ContactParams/1 -> Demux1/1
  Demux1/1 -> Vehicle Local to World/1(State)
  Demux1/3 -> Demux2/1
  Subsystem/1(Out1) -> For All Wheel Contacts/1(In1)
  For All Wheel Contacts/1(Out1) -> Demux/1

== system LMS_cs_old/BMW_X5_SUV_6/SELF_Demux ==
  SELF : Inport  OutDataTypeStr=Bus: PRESCAN_SELFSENSORDATA
  Bus Selector : BusSelector  OutputSignals=PositionX,PositionY,PositionZ,OrientationRoll,OrientationPitch,OrientationYaw,Velocity,Yaw_rate,Lat,Long,Alt
  Demux2 : Demux  Outputs=3
  Gain : Gain  Gain=180/pi
  Gain1 : Gain  Gain=180/pi
  Vector Concatenate1 : Concatenate  NumInputs=3
  compas converter : Subsystem
  x [m] : Outport
  y [m] : Outport  Port=2
  z [m] : Outport  Port=3
  rotx [deg] : Outport  Port=4
  roty [deg] : Outport  Port=5
  rotz [deg] : Outport  Port=6
  GPS lat [deg] : Outport  Port=7
  GPS long [deg] : Outport  Port=8
  GPS alt [m] : Outport  Port=9
  velocity [m/s] : Outport  Port=10
  heading [deg] : Outport  Port=11
  yaw rate [deg/s] : Outport  Port=12
  wires:
  Bus Selector/11 -> GPS alt [m]/1  "<Alt>"
  Bus Selector/10 -> GPS long [deg]/1  "<Long>"
  Bus Selector/9 -> GPS lat [deg]/1  "<Lat>"
  Bus Selector/8 -> Gain1/1  "<Yaw_rate>"
  Bus Selector/7 -> velocity [m/s]/1  "<Velocity>"
  Bus Selector/6 -> compas converter/1(rotz [rad]), Vector Concatenate1/3  "<OrientationYaw>"
  Bus Selector/5 -> Vector Concatenate1/2  "<OrientationPitch>"
  Bus Selector/4 -> Vector Concatenate1/1  "<OrientationRoll>"
  Vector Concatenate1/1 -> Gain/1
  Bus Selector/3 -> z [m]/1  "<PositionZ>"
  Bus Selector/2 -> y [m]/1  "<PositionY>"
  Bus Selector/1 -> x [m]/1  "<PositionX>"
  SELF/1 -> Bus Selector/1
  Gain/1 -> Demux2/1
  Demux2/1 -> rotx [deg]/1
  Demux2/2 -> roty [deg]/1
  Demux2/3 -> rotz [deg]/1
  compas converter/1(heading [deg]) -> heading [deg]/1
  Gain1/1 -> yaw rate [deg/s]/1

== system LMS_cs_old/BMW_X5_SUV_6/STATE_BMW_X5_SUV_6 ==
  State : Inport  SampleTime=TimeStep
  Bus Creator : BusCreator  Inputs=15  OutDataTypeStr=Bus: PRESCAN_STATEACTUATORDATA  NonVirtualBus=on
  Demux : Demux  Outputs=15
  iniBODYAngles wrtVEH [rad] : Constant  Value=[Roll0 Pitch0 0]  SampleTime=TimeStep
  iniVEHAngles wrtGLOB [rad] : Constant  Value=[0 0 Yaw0]  SampleTime=TimeStep
  iniVEHposition wrtGLOB [m] : Constant  Value=[x0 y0 z0]  SampleTime=TimeStep
  state2FullState : PreScanSimulinkLibrary/state2FullState  SystemSampleTime=-1  VariantActivationTime=update diagram  Latency=0  AutoFrameSizeCalculation=off
  StateBus : Outport  OutDataTypeStr=Bus: PRESCAN_STATEACTUATORDATA
  wires:
  Bus Creator/1 -> StateBus/1
  State/1 -> state2FullState/1
  state2FullState/1 -> Demux/1
  iniVEHposition wrtGLOB [m]/1 -> state2FullState/2
  iniBODYAngles wrtVEH [rad]/1 -> state2FullState/3
  iniVEHAngles wrtGLOB [rad]/1 -> state2FullState/4
  Demux/1 -> Bus Creator/1  "PositionX"
  Demux/2 -> Bus Creator/2  "PositionY"
  Demux/3 -> Bus Creator/3  "PositionZ"
  Demux/4 -> Bus Creator/4  "VelocityX"
  Demux/5 -> Bus Creator/5  "VelocityY"
  Demux/6 -> Bus Creator/6  "VelocityZ"
  Demux/7 -> Bus Creator/7  "AccelerationX"
  Demux/8 -> Bus Creator/8  "AccelerationY"
  Demux/9 -> Bus Creator/9  "AccelerationZ"
  Demux/10 -> Bus Creator/10  "OrientationRoll"
  Demux/11 -> Bus Creator/11  "OrientationPitch"
  Demux/12 -> Bus Creator/12  "OrientationYaw"
  Demux/13 -> Bus Creator/13  "AngularVelocityRoll"
  Demux/14 -> Bus Creator/14  "AngularVelocityPitch"
  Demux/15 -> Bus Creator/15  "AngularVelocityYaw"

== system LMS_cs_old/BMW_X5_SUV_6/WheelDisplacement_Mux ==
  Steering Angle Front [rad] : Inport  Tag=inport/JointGroup  SampleTime=2/200  BusOutputAsStruct=on
  Steering Angle Rear [rad] : Inport  Tag=inport/JointGroup  Port=2  SampleTime=2/200  BusOutputAsStruct=on
  Rotation [rad] : Inport  Tag=inport/JointGroup  Port=3  SampleTime=2/200  BusOutputAsStruct=on
  zDisp FL [m] : Inport  Tag=inport/JointGroup  Port=4  SampleTime=2/200  BusOutputAsStruct=on
  zDisp FR [m] : Inport  Tag=inport/JointGroup  Port=5  SampleTime=2/200  BusOutputAsStruct=on
  zDisp RL [m] : Inport  Tag=inport/JointGroup  Port=6  SampleTime=2/200  BusOutputAsStruct=on
  zDisp RR [m] : Inport  Tag=inport/JointGroup  Port=7  SampleTime=2/200  BusOutputAsStruct=on
  Ground_{1..12} (12 alike) : Ground
  WheelL0_Mux : Subsystem  Tag=mux/Joint  mask(PreScan Mux Block){DisplayName=WheelL0}
      mask prompts: DisplayName "Display Name"
      mask help:
      | This block simulates a generic joint used for generic models. This joint can be enabled/disabled from the GUI.
      |
      | For more information, please click Help.
      settings: DeleteFcn=PreScanBlockDeleteFcn;
      mask Help: eval('openHelp(254)')
  WheelL1_Mux : Subsystem  Tag=mux/Joint  mask(PreScan Mux Block){DisplayName=WheelL1}
      mask prompts: DisplayName "Display Name"
      mask help:
      | This block simulates a generic joint used for generic models. This joint can be enabled/disabled from the GUI.
      |
      | For more information, please click Help.
      settings: DeleteFcn=PreScanBlockDeleteFcn;
      mask Help: eval('openHelp(254)')
  WheelR0_Mux : Subsystem  Tag=mux/Joint  mask(PreScan Mux Block){DisplayName=WheelR0}
      mask prompts: DisplayName "Display Name"
      mask help:
      | This block simulates a generic joint used for generic models. This joint can be enabled/disabled from the GUI.
      |
      | For more information, please click Help.
      settings: DeleteFcn=PreScanBlockDeleteFcn;
      mask Help: eval('openHelp(254)')
  WheelR1_Mux : Subsystem  Tag=mux/Joint  mask(PreScan Mux Block){DisplayName=WheelR1}
      mask prompts: DisplayName "Display Name"
      mask help:
      | This block simulates a generic joint used for generic models. This joint can be enabled/disabled from the GUI.
      |
      | For more information, please click Help.
      settings: DeleteFcn=PreScanBlockDeleteFcn;
      mask Help: eval('openHelp(254)')
  WheelL0_BMW_X5_SUV_6 : Outport  Tag=outport/JointActuator  OutDataTypeStr=Bus: PRESCAN_POSE_DATA  SampleTime=2/200
  WheelR0_BMW_X5_SUV_6 : Outport  Tag=outport/JointActuator  Port=2  OutDataTypeStr=Bus: PRESCAN_POSE_DATA  SampleTime=2/200
  WheelR1_BMW_X5_SUV_6 : Outport  Tag=outport/JointActuator  Port=3  OutDataTypeStr=Bus: PRESCAN_POSE_DATA  SampleTime=2/200
  WheelL1_BMW_X5_SUV_6 : Outport  Tag=outport/JointActuator  Port=4  OutDataTypeStr=Bus: PRESCAN_POSE_DATA  SampleTime=2/200
  wires:
  WheelL0_Mux/1(Joint) -> WheelL0_BMW_X5_SUV_6/1
  WheelR0_Mux/1(Joint) -> WheelR0_BMW_X5_SUV_6/1
  WheelR1_Mux/1(Joint) -> WheelR1_BMW_X5_SUV_6/1
  WheelL1_Mux/1(Joint) -> WheelL1_BMW_X5_SUV_6/1
  Steering Angle Front [rad]/1 -> WheelR0_Mux/6(Yaw [rad]), WheelL0_Mux/6(Yaw [rad])
  Steering Angle Rear [rad]/1 -> WheelR1_Mux/6(Yaw [rad]), WheelL1_Mux/6(Yaw [rad])
  Rotation [rad]/1 -> WheelR0_Mux/5(Pitch [rad]), WheelL0_Mux/5(Pitch [rad]), WheelR1_Mux/5(Pitch [rad]), WheelL1_Mux/5(Pitch [rad])
  zDisp FL [m]/1 -> WheelL0_Mux/3(Z [m])
  zDisp FR [m]/1 -> WheelR0_Mux/3(Z [m])
  zDisp RL [m]/1 -> WheelL1_Mux/3(Z [m])
  zDisp RR [m]/1 -> WheelR1_Mux/3(Z [m])
  Ground_1/1 -> WheelL0_Mux/1(X [m])
  Ground_2/1 -> WheelL0_Mux/2(Y [m])
  Ground_3/1 -> WheelL0_Mux/4(Roll [rad])
  Ground_4/1 -> WheelL1_Mux/1(X [m])
  Ground_5/1 -> WheelL1_Mux/2(Y [m])
  Ground_6/1 -> WheelL1_Mux/4(Roll [rad])
  Ground_7/1 -> WheelR0_Mux/1(X [m])
  Ground_8/1 -> WheelR0_Mux/2(Y [m])
  Ground_9/1 -> WheelR0_Mux/4(Roll [rad])
  Ground_10/1 -> WheelR1_Mux/1(X [m])
  Ground_11/1 -> WheelR1_Mux/2(Y [m])
  Ground_12/1 -> WheelR1_Mux/4(Roll [rad])

== system LMS_cs_old/BMW_X5_SUV_7/Dynamics_Simple_3D ==
  DeltaSteer_[deg] : Inport
  Throttle : Inport  Port=2
  Brake : Inport  Port=3
  Initial_Vx_[ms-1] : Inport  Port=4
  AutoManual_OnOff : Inport  Port=5
  Auto_GearShift : Inport  Port=6
  Manual_GearShift : Inport  Port=7
  TyreInfo_in : Inport  Port=8
  Bus Creator : BusCreator  Inputs=14
  Bus Selector : BusSelector  OutputSignals=z_wheelFL_[m],z_wheelFR_[m],z_wheelRL_[m],z_wheelRR_[m]
  Chassis : Subsystem
      mask Display: image(imread('Chassis.png'));
  Engine : Subsystem
      mask Display: image(imread('Engine.png'));
  Gain : Gain  Gain=3.6
  Gear: Auto Manual : Subsystem
  Mux : Mux  Inputs=3
  Radians to Degrees : simulink_extras/Transformations/Radians to Degrees
  Radians to Degrees1 : simulink_extras/Transformations/Radians to Degrees
  Selector : Selector  InputPortWidth=9  IndexOptions=Index vector (dialog)  Indices=7  OutputSizes=1
  Selector1 : Selector  InputPortWidth=9  IndexOptions=Index vector (dialog)  Indices=8  OutputSizes=1
  ShiftLogic : Subsystem
      mask Display: image(imread('Gearshift.png'));
  Transmission : Subsystem
      mask Display: image(imread('Transmission.png'));
  State : Outport
  Vx [m s-1] : Outport  Port=2
  Perf_Params : Outport  Port=3
  z_wheelFL_[m] : Outport  Port=4
  z_wheelFR_[m] : Outport  Port=5
  z_wheelRL_[m] : Outport  Port=6
  z_wheelRR_[m] : Outport  Port=7
  ContactParams : Outport  Port=8
  wires:
  [ax] -> Bus Creator/4  "Ax_[ms-2]"
  [vx] -> Gain/1
  Selector1/1 -> Radians to Degrees1/1
  Selector/1 -> Radians to Degrees/1
  [PD] -> Bus Creator/10  "PDrive_[kW]"
  Radians to Degrees1/1 -> Bus Creator/12  "Pitch_[deg]"
  Radians to Degrees/1 -> Bus Creator/11  "Roll_[deg]"
  [PE] -> Bus Creator/9  "PEngine_[kW]"
  Bus Creator/1 -> Perf_Params/1
  Engine/2(PEngine_[kW]) -> [PE]
  [brake] -> Bus Creator/8  "Brake_[bar]"
  [throttle] -> Bus Creator/7  "Throttle_[perc]"
  [auto_manual] -> Bus Creator/6  "Auto_Manual_[-]"
  [ay] -> Bus Creator/5  "Ay_[ms-2]"
  [gear] -> Bus Creator/3  "Gear_[-]"
  [RPM] -> Bus Creator/2  "NEngine_[rpm]"
  Gain/1 -> Bus Creator/1  "Vx_[kmh-1]"
  Transmission/1(ImpellerTorque_[Nm]) -> Engine/1(ImpellerTorque_[Nm])  "ImpellerTorque_[Nm]"
  Transmission/2(TransmissionTorque_[Nm]) -> Chassis/1(TransmissionTorque_[Nm])  "TransmissionTorque_[Nm]"
  ShiftLogic/1(GearNr) -> ShiftLogic/2(GearNr_[-]), Gear: Auto Manual/3(Auto_Gear)  "GearNr_[-]"
  Engine/1(nEngine_[rpm]) -> Transmission/1(nEngine_[rpm]), [RPM]  "nEngine_[rpm]"
  Chassis/1(State) -> Selector1/1, Selector/1, State/1, Mux/1
  DeltaSteer_[deg]/1 -> Chassis/3(DeltaSteer_[deg])
  Initial_Vx_[ms-1]/1 -> Chassis/4(Initial_Vx_[ms-1])
  Throttle/1 -> [throttle], ShiftLogic/1(Throttle_[%]), Engine/2(Throttle_[%])
  Auto_GearShift/1 -> ShiftLogic/3(Auto_GearShift)
  Chassis/7(TransmissionOut_[rpm]) -> Transmission/3(n_TransmissionOut_[rpm])  "n_driveline_[rpm]"
  Chassis/2(VehicleSpeed_[ms-1]) -> [vx], Vx [m s-1]/1, Mux/2  "vx_[ms-1]"
  AutoManual_OnOff/1 -> [auto_manual], Gear: Auto Manual/1(Auto_Manual)
  Manual_GearShift/1 -> Gear: Auto Manual/2(Manual_Gear)
  Gear: Auto Manual/1(Gear) -> [gear], Transmission/2(GearNr_[-])  "gear"
  [vx] -> ShiftLogic/4(VehSpeed_[ms-1])
  TyreInfo_in/1 -> Chassis/5(TyreInfo_in)
  Brake/1 -> Chassis/2(BrakePressure_[bar]), [brake]
  Chassis/6(PDrive_[kW]) -> [PD]
  Chassis/5(ay_[ms-2]) -> [ay]
  Chassis/4(ax_[ms-2]) -> [ax]
  Chassis/3(Vy_[ms-1]) -> [vy]
  [vx] -> Bus Creator/13  "vx_[ms-1]"
  [vy] -> Bus Creator/14  "vy_[ms-1]"
  Chassis/8(z_wheel_[m]) -> Bus Selector/1, Mux/3  "z_wheel_[m]"
  Bus Selector/1 -> z_wheelFL_[m]/1  "<z_wheelFL_[m]>"
  Bus Selector/2 -> z_wheelFR_[m]/1  "<z_wheelFR_[m]>"
  Bus Selector/3 -> z_wheelRL_[m]/1  "<z_wheelRL_[m]>"
  Bus Selector/4 -> z_wheelRR_[m]/1  "<z_wheelRR_[m]>"
  Mux/1 -> ContactParams/1

== system LMS_cs_old/BMW_X5_SUV_7/JointGroup_WheelDisplacement_V2R ==
  Velocity [m/s] : Inport  SampleTime=TimeStep
  Discrete-Time Integrator : DiscreteIntegrator  SampleTime=TimeStep  ICPrevOutput=DiscIntNeverNeededParam  ICPrevScaledInput=DiscIntNeverNeededParam
  omega=V/Rwheel : Gain  Gain=1/TireRadius
  Rotation [rad] : Outport
  wires:
  Discrete-Time Integrator/1 -> Rotation [rad]/1  "roty"
  omega=V/Rwheel/1 -> Discrete-Time Integrator/1  "rotational speed [rad/s]"
  Velocity [m/s]/1 -> omega=V/Rwheel/1

== system LMS_cs_old/BMW_X5_SUV_7/PreScan_Contact_Sensor ==
  ContactParams : Inport  SampleTime=TimeStep
  Steer Angle Front [deg] : Inport  Port=2
  Steer Angle Rear [deg] : Inport  Port=3
  Bus Creator2 : BusCreator  Inputs=4
  Demux : Demux
  Demux1 : Demux  Outputs=[9 1 4]
  Demux2 : Demux
  For All Wheel Contacts : Subsystem  TreatAsAtomicUnit=on
  Mux6 : Mux  Inputs=2
  Subsystem : Subsystem  mask{NumberOfWheels=4, MaxContactPoints=4, WheelRadius=wheelRadius, WheelWidth=0.2}
      mask prompts: NumberOfWheels "Number of Wheels"; MaxContactPoints "Maximum number of Contact Points"; WheelRadius "Wheel Radius"; WheelWidth "Wheel Width"
      mask Display: disp('Contact Sensor')
  Tire Collision Demux : Subsystem
  Tire Collision Demux1 : Subsystem
  Tire Collision Demux2 : Subsystem
  Tire Collision Demux3 : Subsystem
  Vehicle Local to World : Subsystem
  Wheels = 4 : Subsystem  mask{NumberOfWheels=4}
      mask prompts: NumberOfWheels "Number of Wheels"
      mask Display:
      | port_label('input', 1,'Vehicle wrt World')
      | port_label('input', 2,'Wheels wrt World')
  Wheels Local to World : Subsystem  Tag=MuxWheels  mask(PreScan Mux Block:){}
      settings: DeleteFcn=PreScanBlockDeleteFcn;
  Results : Outport
  wires:
  Mux6/1 -> Wheels = 4/1(Vehicle wrt World)
  Wheels = 4/1(WheelPoses) -> Subsystem/1(In1)
  Demux/1 -> Tire Collision Demux/1(demux in)
  Demux/2 -> Tire Collision Demux1/1(demux in)
  Demux/3 -> Tire Collision Demux2/1(demux in)
  Demux/4 -> Tire Collision Demux3/1(demux in)
  Tire Collision Demux/1(bus out) -> Bus Creator2/1  "TireFL"
  Tire Collision Demux1/1(bus out) -> Bus Creator2/2  "TireFR"
  Tire Collision Demux2/1(bus out) -> Bus Creator2/3  "TireRL"
  Tire Collision Demux3/1(bus out) -> Bus Creator2/4  "TireRR"
  Vehicle Local to World/1(Position) -> Mux6/1
  Vehicle Local to World/2(Orientation) -> Mux6/2
  Wheels Local to World/1(Wheel Poses) -> Wheels = 4/2(Wheels wrt World)
  Demux1/2 -> Wheels Local to World/3(Velocity [m/s])
  Demux2/1 -> Wheels Local to World/4(zDisp FL [m])
  Demux2/2 -> Wheels Local to World/5(zDisp FR [m])
  Demux2/3 -> Wheels Local to World/6(zDisp RL [m])
  Demux2/4 -> Wheels Local to World/7(zDisp RR [m])
  Steer Angle Front [deg]/1 -> Wheels Local to World/1(Steer Angle Front [deg])
  Steer Angle Rear [deg]/1 -> Wheels Local to World/2(Steer Angle Rear [deg])
  Bus Creator2/1 -> Results/1
  ContactParams/1 -> Demux1/1
  Demux1/1 -> Vehicle Local to World/1(State)
  Demux1/3 -> Demux2/1
  Subsystem/1(Out1) -> For All Wheel Contacts/1(In1)
  For All Wheel Contacts/1(Out1) -> Demux/1
